simulink model "ART25_full_car_old"  (R2022a)
settings: Solver=ode1  StartTime=1  StopTime=10  FixedStep=0.0001  RelTol=1e-3
undefined symbols (not defined in the file or in its folder): canChannel, param, sim_TimeStep, vx0, yaw_rate0
libraries: canmsglib x5, slpidlib x4, canlib x2
settings Model: PacingRate=0.200000  Creator=jutri  LastModifiedBy=Usuario
settings SolverCC: PositivePriorityOrder=on
settings DataIOCC: SaveFormat=Array
settings OptimizationCC: BlockReduction=off  OptimizeBlockIOStorage=off
settings DebuggingCC: TasksWithSamePriorityMsg=none
settings HardwareCC: ProdBitPerLong=64  ProdHWDeviceType=Intel->x86-64 (Linux 64)
settings ModelReferenceCC: EnableRefExpFcnMdlSchedulingChecks=off  ModelReferenceNumInstancesAllowed=Single
settings RTWCC: Description=Simulink Desktop Real-Time  SystemTargetFile=sldrt.tlc  TemplateMakefile=sldrt.tmf  Toolchain=Simulink Real-Time Toolchain  BuildConfiguration=Faster Runs  TargetLang=C++  RTWCompilerOptimization=on
settings CodeAppCC: MaxIdLength=95
settings SimulinkDesktopRealTimeCC: TargetLibSuffix=_sldrt.a  TargetPreCompLibLocation=C:\Program Files\MATLAB\R2022a\toolbox\sldrt\lib\win64  TargetLangStandard=C++03 (ISO)

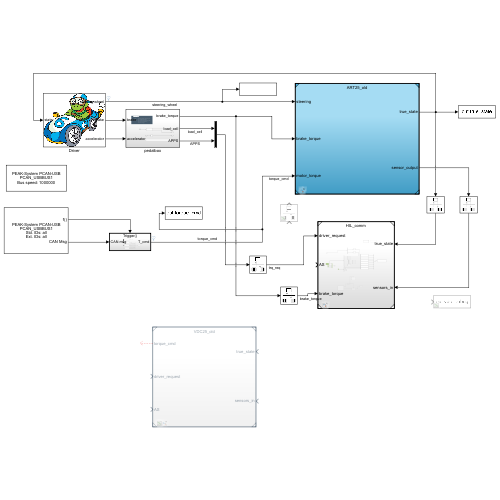
[thumbnail: Simulink's stored preview of the top-level diagram]
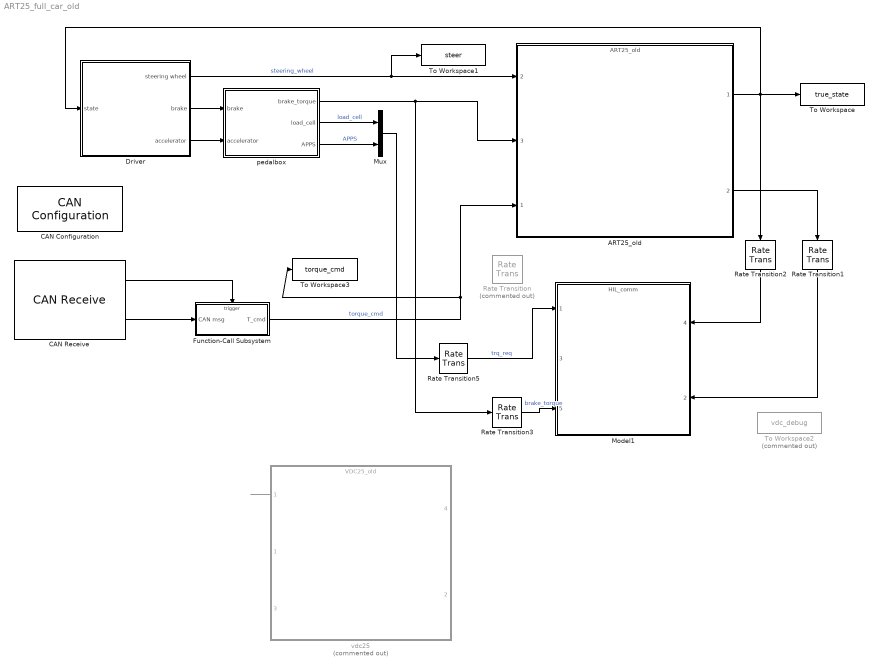
== system ART25_full_car_old ==
  ART25_old : ModelReference  ModelNameDialog=ART25_old.slx  SimulationMode=Normal  ModelReferenceVersion=1.103
      settings: PortSchema="{\"entries\":[{\"content\":{\"sides\":[{\"content\":{\"connectorIds\":[\"In2\",\"In3\",\"In1\"]},\"type\":\"ConnectorPlacement.EquallySpacedRectSide\",\"uuid\":\"34e73162-f48c-446a-824e-17dcc9cc6514\"},{\"content\":{\"connectorIds\":[\"Out1\",\"Out2\"],\"side\":\"RIGHT\"},\"type\":\"ConnectorPlacement.EquallySpacedRectSide\",\"uuid\":\"74737ed4-0958-463a-8e43-c11e4d3189aa\"},{\"content\":{\"side\":\"TOP\"},\"type\":\"ConnectorPlacement.EquallySpacedRectSide\",\"uuid\":\"42fc3775-e72e-4fbb-8cdc-9d9cf3c0f815\"}]},\"type\":\"ConnectorPlacement.EquallySpacedConnector\",\"uuid\":\"6e643428-a593-4a05-90a3-6bfae895b914\"}],\"packageUris\":[\"http://schema.mathworks.com/mf0/Connector/R2020b\"],\"version\":\"1.0\"}"
  CAN Configuration : canlib/CAN Configuration  BlockHandle=8.0004  Device=PEAK-System PCAN-USB (PCAN_USBBUS1)  DeviceMenu=PEAK-System PCAN-USB (PCAN_USBBUS1)  ObjConstructor=canChannel('PEAK-System', 'PCAN_USBBUS1')  BusSpeed=1000000  EnableBitParameters=off  AckMode=Normal
      settings: SourceProductBaseCode=VN
  CAN Receive : canlib/CAN Receive  BlockHandle=9.0004  Device=PEAK-System PCAN-USB (PCAN_USBBUS1)  DeviceMenu=PEAK-System PCAN-USB (PCAN_USBBUS1)  ObjConstructor=canChannel('PEAK-System', 'PCAN_USBBUS1')  EnableStandardIDsFilter=off  StdIDsCombo=Allow all  StandardIDs=0  EnableExtendedIDsFilter=off  ExtIDsCombo=Allow all  ExtendedIDs=0  SampleTime=sim_TimeStep  MsgsPerTimestep=all  InternalFilterUpdateStatus=on  BusOutput=off
      settings: SourceProductBaseCode=VN
  Driver : Subsystem
      mask Display: image('Driver_logo.jpeg');
  Function-Call Subsystem : Subsystem  TreatAsAtomicUnit=on
  Model1 : ModelReference  ModelNameDialog=HIL_comm.slx  SimulationMode=Normal  ModelReferenceVersion=1.270
      settings: PortSchema="{\"entries\":[{\"content\":{\"sides\":[{\"content\":{\"connectorIds\":[\"In1\",\"In3\",\"In5\"]},\"type\":\"ConnectorPlacement.EquallySpacedRectSide\",\"uuid\":\"04602d22-b9d7-40f7-b052-73f4143762fc\"},{\"content\":{\"connectorIds\":[\"In4\",\"In2\"],\"side\":\"RIGHT\"},\"type\":\"ConnectorPlacement.EquallySpacedRectSide\",\"uuid\":\"c5daacf6-0ad1-4531-a33a-b3ee5e66ed07\"},{\"content\":{\"connectorIds\":[],\"side\":\"TOP\"},\"type\":\"ConnectorPlacement.EquallySpacedRectSide\",\"uuid\":\"aa04230c-105f-45b7-b831-453931269445\"}]},\"type\":\"ConnectorPlacement.EquallySpacedConnector\",\"uuid\":\"55928aa8-a510-4f66-80b8-414931ecc3aa\"}],\"packageUris\":[\"http://schema.mathworks.com/mf0/Connector/R2020b\"],\"version\":\"1.0\"}"
  Mux : Mux  Inputs=2
  Rate Transition : RateTransition  Commented=on
  Rate Transition1 : RateTransition  Deterministic=off  OutPortSampleTime=vdc_TimeStep
  Rate Transition2 : RateTransition  OutPortSampleTime=vdc_TimeStep
  Rate Transition3 : RateTransition  OutPortSampleTime=vdc_TimeStep
  Rate Transition5 : RateTransition  OutPortSampleTime=vdc_TimeStep
  To Workspace : ToWorkspace  VariableName=true_state  SaveFormat=Structure With Time  SampleTime=-1
  To Workspace1 : ToWorkspace  VariableName=steer  SaveFormat=Structure  SampleTime=-1
  To Workspace2 : ToWorkspace  Commented=on  VariableName=vdc_debug  SaveFormat=Structure With Time  SampleTime=-1
  To Workspace3 : ToWorkspace  VariableName=torque_cmd  SaveFormat=Structure With Time  SampleTime=-1
  pedalbox : Subsystem
  vdc25 : ModelReference  Commented=on  ModelNameDialog=VDC25_old.slx  SimulationMode=Normal  ModelReferenceVersion=1.159
      settings: PortSchema="{\"entries\":[{\"content\":{\"sides\":[{\"content\":{\"connectorIds\":[\"Out1\",\"In1\",\"In3\"]},\"type\":\"ConnectorPlacement.EquallySpacedRectSide\",\"uuid\":\"da147370-b91a-4bb5-9c6b-40685e9dd617\"},{\"content\":{\"connectorIds\":[\"In4\",\"In2\"],\"side\":\"RIGHT\"},\"type\":\"ConnectorPlacement.EquallySpacedRectSide\",\"uuid\":\"d61eec38-a682-4bd1-95e6-e7fb713ea16a\"},{\"content\":{\"connectorIds\":[],\"side\":\"TOP\"},\"type\":\"ConnectorPlacement.EquallySpacedRectSide\",\"uuid\":\"c636197e-c055-4dae-9ca6-30a202bee6bf\"}]},\"type\":\"ConnectorPlacement.EquallySpacedConnector\",\"uuid\":\"636ba342-8237-45ef-8445-7b2704fdba3c\"}],\"packageUris\":[\"http://schema.mathworks.com/mf0/Connector/R2020b\"],\"version\":\"1.0\"}"
  wires:
  Driver/1(steering wheel) -> To Workspace1/1, ART25_old/2  "steering_wheel"
  ART25_old/2 -> Rate Transition1/1
  Driver/2(brake) -> pedalbox/1(brake)
  vdc25/1 -> ?
  ART25_old/1 -> Driver/1(state), Rate Transition2/1, To Workspace/1
  Driver/3(accelerator) -> pedalbox/2(accelerator)
  pedalbox/2(load_cell) -> Mux/1  "load_cell"
  pedalbox/3(APPS) -> Mux/2  "APPS"
  Rate Transition5/1 -> Model1/1  "trq_req"
  Rate Transition1/1 -> Model1/2
  Rate Transition2/1 -> Model1/4
  Mux/1 -> Rate Transition5/1
  CAN Receive/2 -> Function-Call Subsystem/1(CAN msg)
  CAN Receive/1 -> Function-Call Subsystem/Trigger
  Function-Call Subsystem/1(T_cmd) -> ART25_old/1, To Workspace3/1  "torque_cmd"
  Rate Transition3/1 -> Model1/5  "brake_torque"
  pedalbox/1(brake_torque) -> Rate Transition3/1, ART25_old/3

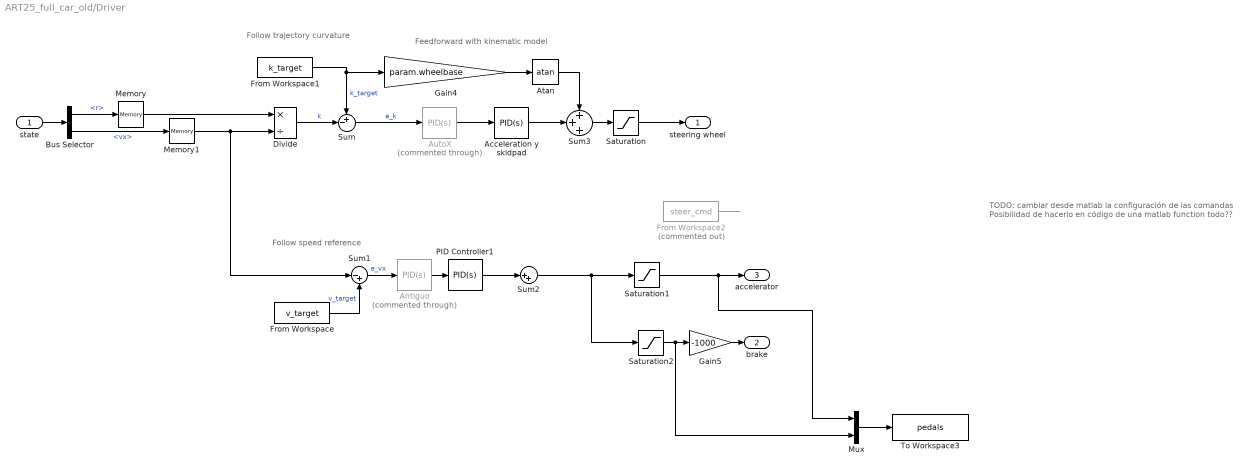
== system ART25_full_car_old/Driver ==
  note: TODO: cambiar desde matlab la configuración de las comandas
      | Posibilidad de hacerlo en código de una matlab function todo??
  note: Feedforward with kinematic model
  note: Follow trajectory curvature
  note: Follow speed reference
  state : Inport
  Acceleration y skidpad : slpidlib/PID Controller  Controller=PID  Form=Parallel  TimeDomain=Continuous-time  UseExternalTs=off  SampleTime=-1  IntegratorMethod=Forward Euler  FilterMethod=Forward Euler  ControllerParametersSource=internal  P=1  I=5  UseKiTs=off  D=0  N=1  UseFilter=on  TunerSelectOption=Transfer Function Based (PID Tuner App)  InitialConditionSource=internal  InitialConditionForIntegrator=0  InitialConditionForFilter=0  DifferentiatorICPrevScaledInput=0  ExternalReset=none  TrackingMode=off  Kt=1  LimitOutput=off  SatLimitsSource=internal  UpperSaturationLimit=inf  LowerSaturationLimit=-inf  LinearizeAsGain=on  AntiWindupMode=none  Kb=1  POutMin=[]  POutMax=[]  IOutMin=[]  IOutMax=[]  DOutMin=[]  DOutMax=[]  NOutMin=[]  NOutMax=[]  SumOutMin=[]  SumOutMax=[]  SaturationOutMin=[]  SaturationOutMax=[]  PParamMin=[]  PParamMax=[]  IParamMin=[]  IParamMax=[]  DParamMin=[]  DParamMax=[]  NParamMin=[]  NParamMax=[]  KbParamMin=[]  KbParamMax=[]  KtParamMin=[]  KtParamMax=[]  KbOutMin=[]  KbOutMax=[]  KtOutMin=[]  KtOutMax=[]  IntegratorOutMin=[]  IntegratorOutMax=[]  FilterOutMin=[]  FilterOutMax=[]  SumI1OutMin=[]  SumI1OutMax=[]  SumI2OutMin=[]  SumI2OutMax=[]  SumI3OutMin=[]  SumI3OutMax=[]  SumI4OutMin=[]  SumI4OutMax=[]  SumDOutMin=[]  SumDOutMax=[]  DifferentiatorOutMin=[]  DifferentiatorOutMax=[]  FilterDiffOutCoefMin=[]  FilterDiffOutCoefMax=[]  ReciprocalOutMin=[]  ReciprocalOutMax=[]  SumDenOutMin=[]  SumDenOutMax=[]  SumNumOutMin=[]  SumNumOutMax=[]  DivideOutMin=[]  DivideOutMax=[]  UdiffTsProdOutMin=[]  UdiffTsProdOutMax=[]  NTsProdOutMin=[]  NTsProdOutMax=[]  UintegralTsProdOutMin=[]  UintegralTsProdOutMax=[]  UngainTsProdOutMin=[]  UngainTsProdOutMax=[]  ClampingZeroOutDataTypeStr=Inherit: Inherit via back propagation  ClampingZeroOutMin=[]  ClampingZeroOutMax=[]  FilterDenConstantOutDataTypeStr=Inherit: Inherit via back propagation  FilterDenConstantOutMin=[]  FilterDenConstantOutMax=[]  PCopyOutDataTypeStr=Inherit: Inherit via back propagation  PCopyOutMin=[]  PCopyOutMax=[]  NCopyOutDataTypeStr=Inherit: Inherit via back propagation  NCopyOutMin=[]  NCopyOutMax=[]  IntegratorContinuousStateAttributes=''  IntegratorStateMustResolveToSignalObject=off  IntegratorRTWStateStorageClass=Auto  FilterContinuousStateAttributes=''  FilterStateMustResolveToSignalObject=off  FilterRTWStateStorageClass=Auto  ParallelPVariant=InternalParameters  IdealPVariant=Disabled  IVariant=InternalParameters  DVariant=InternalParameters  IntegratorVariant=Continuous  SatVariant=Disabled  AWVariant=Passthrough  PCopyVariant=Disabled  TRVariant=Disabled  FdbkBlocksVariant=Forward  IdealPFdbkVariant=Disabled  SatFdbkVariant=Disabled  DerivativeFilterVariant=ContFilter  NVariant=InternalParameters  NCopyVariant=Disabled  FilterICVariant=InternalICsFilter  IntegratorICVariant=InternalICs  ExternalResetVariant=Disabled  TRSumVariant=Passthrough  SumFdbkVariant=Disabled  SumVariant=Sum_PID  TsampFilterVariant=InternalTs  TsampNgainVariant=Passthrough  TsampIntegralVariant=Passthrough  ExternalSaturationOutDataTypeStr=Inherit: Same as second input  aMode=0
  Antiguo : slpidlib/PID Controller  Commented=through  Controller=PID  Form=Parallel  TimeDomain=Continuous-time  UseExternalTs=off  SampleTime=-1  IntegratorMethod=Forward Euler  FilterMethod=Forward Euler  ControllerParametersSource=internal  P=1  I=1  UseKiTs=off  D=0  N=10  UseFilter=on  TunerSelectOption=Transfer Function Based (PID Tuner App)  InitialConditionSource=internal  InitialConditionForIntegrator=0  InitialConditionForFilter=0  DifferentiatorICPrevScaledInput=0  ExternalReset=none  TrackingMode=off  Kt=1  LimitOutput=off  SatLimitsSource=internal  UpperSaturationLimit=inf  LowerSaturationLimit=-inf  LinearizeAsGain=on  AntiWindupMode=none  Kb=1  POutMin=[]  POutMax=[]  IOutMin=[]  IOutMax=[]  DOutMin=[]  DOutMax=[]  NOutMin=[]  NOutMax=[]  SumOutMin=[]  SumOutMax=[]  SaturationOutMin=[]  SaturationOutMax=[]  PParamMin=[]  PParamMax=[]  IParamMin=[]  IParamMax=[]  DParamMin=[]  DParamMax=[]  NParamMin=[]  NParamMax=[]  KbParamMin=[]  KbParamMax=[]  KtParamMin=[]  KtParamMax=[]  KbOutMin=[]  KbOutMax=[]  KtOutMin=[]  KtOutMax=[]  IntegratorOutMin=[]  IntegratorOutMax=[]  FilterOutMin=[]  FilterOutMax=[]  SumI1OutMin=[]  SumI1OutMax=[]  SumI2OutMin=[]  SumI2OutMax=[]  SumI3OutMin=[]  SumI3OutMax=[]  SumI4OutMin=[]  SumI4OutMax=[]  SumDOutMin=[]  SumDOutMax=[]  DifferentiatorOutMin=[]  DifferentiatorOutMax=[]  FilterDiffOutCoefMin=[]  FilterDiffOutCoefMax=[]  ReciprocalOutMin=[]  ReciprocalOutMax=[]  SumDenOutMin=[]  SumDenOutMax=[]  SumNumOutMin=[]  SumNumOutMax=[]  DivideOutMin=[]  DivideOutMax=[]  UdiffTsProdOutMin=[]  UdiffTsProdOutMax=[]  NTsProdOutMin=[]  NTsProdOutMax=[]  UintegralTsProdOutMin=[]  UintegralTsProdOutMax=[]  UngainTsProdOutMin=[]  UngainTsProdOutMax=[]  ClampingZeroOutDataTypeStr=Inherit: Inherit via back propagation  ClampingZeroOutMin=[]  ClampingZeroOutMax=[]  FilterDenConstantOutDataTypeStr=Inherit: Inherit via back propagation  FilterDenConstantOutMin=[]  FilterDenConstantOutMax=[]  PCopyOutDataTypeStr=Inherit: Inherit via back propagation  PCopyOutMin=[]  PCopyOutMax=[]  NCopyOutDataTypeStr=Inherit: Inherit via back propagation  NCopyOutMin=[]  NCopyOutMax=[]  IntegratorContinuousStateAttributes=''  IntegratorStateMustResolveToSignalObject=off  IntegratorRTWStateStorageClass=Auto  FilterContinuousStateAttributes=''  FilterStateMustResolveToSignalObject=off  FilterRTWStateStorageClass=Auto  ParallelPVariant=InternalParameters  IdealPVariant=Disabled  IVariant=InternalParameters  DVariant=InternalParameters  IntegratorVariant=Continuous  SatVariant=Disabled  AWVariant=Passthrough  PCopyVariant=Disabled  TRVariant=Disabled  FdbkBlocksVariant=Forward  IdealPFdbkVariant=Disabled  SatFdbkVariant=Disabled  DerivativeFilterVariant=ContFilter  NVariant=InternalParameters  NCopyVariant=Disabled  FilterICVariant=InternalICsFilter  IntegratorICVariant=InternalICs  ExternalResetVariant=Disabled  TRSumVariant=Passthrough  SumFdbkVariant=Disabled  SumVariant=Sum_PID  TsampFilterVariant=InternalTs  TsampNgainVariant=Passthrough  TsampIntegralVariant=Passthrough  ExternalSaturationOutDataTypeStr=Inherit: Same as second input  aMode=0
  Atan : Trigonometry  Operator=atan
  AutoX : slpidlib/PID Controller  Commented=through  Controller=PID  Form=Parallel  TimeDomain=Continuous-time  UseExternalTs=off  SampleTime=-1  IntegratorMethod=Forward Euler  FilterMethod=Forward Euler  ControllerParametersSource=internal  P=1  I=2  UseKiTs=off  D=0.4  N=500  UseFilter=on  TunerSelectOption=Transfer Function Based (PID Tuner App)  InitialConditionSource=internal  InitialConditionForIntegrator=0  InitialConditionForFilter=0  DifferentiatorICPrevScaledInput=0  ExternalReset=none  TrackingMode=off  Kt=1  LimitOutput=off  SatLimitsSource=internal  UpperSaturationLimit=inf  LowerSaturationLimit=-inf  LinearizeAsGain=on  AntiWindupMode=none  Kb=1  POutMin=[]  POutMax=[]  IOutMin=[]  IOutMax=[]  DOutMin=[]  DOutMax=[]  NOutMin=[]  NOutMax=[]  SumOutMin=[]  SumOutMax=[]  SaturationOutMin=[]  SaturationOutMax=[]  PParamMin=[]  PParamMax=[]  IParamMin=[]  IParamMax=[]  DParamMin=[]  DParamMax=[]  NParamMin=[]  NParamMax=[]  KbParamMin=[]  KbParamMax=[]  KtParamMin=[]  KtParamMax=[]  KbOutMin=[]  KbOutMax=[]  KtOutMin=[]  KtOutMax=[]  IntegratorOutMin=[]  IntegratorOutMax=[]  FilterOutMin=[]  FilterOutMax=[]  SumI1OutMin=[]  SumI1OutMax=[]  SumI2OutMin=[]  SumI2OutMax=[]  SumI3OutMin=[]  SumI3OutMax=[]  SumI4OutMin=[]  SumI4OutMax=[]  SumDOutMin=[]  SumDOutMax=[]  DifferentiatorOutMin=[]  DifferentiatorOutMax=[]  FilterDiffOutCoefMin=[]  FilterDiffOutCoefMax=[]  ReciprocalOutMin=[]  ReciprocalOutMax=[]  SumDenOutMin=[]  SumDenOutMax=[]  SumNumOutMin=[]  SumNumOutMax=[]  DivideOutMin=[]  DivideOutMax=[]  UdiffTsProdOutMin=[]  UdiffTsProdOutMax=[]  NTsProdOutMin=[]  NTsProdOutMax=[]  UintegralTsProdOutMin=[]  UintegralTsProdOutMax=[]  UngainTsProdOutMin=[]  UngainTsProdOutMax=[]  ClampingZeroOutDataTypeStr=Inherit: Inherit via back propagation  ClampingZeroOutMin=[]  ClampingZeroOutMax=[]  FilterDenConstantOutDataTypeStr=Inherit: Inherit via back propagation  FilterDenConstantOutMin=[]  FilterDenConstantOutMax=[]  PCopyOutDataTypeStr=Inherit: Inherit via back propagation  PCopyOutMin=[]  PCopyOutMax=[]  NCopyOutDataTypeStr=Inherit: Inherit via back propagation  NCopyOutMin=[]  NCopyOutMax=[]  IntegratorContinuousStateAttributes=''  IntegratorStateMustResolveToSignalObject=off  IntegratorRTWStateStorageClass=Auto  FilterContinuousStateAttributes=''  FilterStateMustResolveToSignalObject=off  FilterRTWStateStorageClass=Auto  ParallelPVariant=InternalParameters  IdealPVariant=Disabled  IVariant=InternalParameters  DVariant=InternalParameters  IntegratorVariant=Continuous  SatVariant=Disabled  AWVariant=Passthrough  PCopyVariant=Disabled  TRVariant=Disabled  FdbkBlocksVariant=Forward  IdealPFdbkVariant=Disabled  SatFdbkVariant=Disabled  DerivativeFilterVariant=ContFilter  NVariant=InternalParameters  NCopyVariant=Disabled  FilterICVariant=InternalICsFilter  IntegratorICVariant=InternalICs  ExternalResetVariant=Disabled  TRSumVariant=Passthrough  SumFdbkVariant=Disabled  SumVariant=Sum_PID  TsampFilterVariant=InternalTs  TsampNgainVariant=Passthrough  TsampIntegralVariant=Passthrough  ExternalSaturationOutDataTypeStr=Inherit: Same as second input  aMode=0
  Bus Selector : BusSelector  OutputSignals=r,vx
  Divide : Product  Inputs=*/
  From Workspace : FromWorkspace  VariableName=v_target
  From Workspace1 : FromWorkspace  VariableName=k_target
  From Workspace2 : FromWorkspace  Commented=on  VariableName=steer_cmd
  Gain4 : Gain  Gain=param.wheelbase
  Gain5 : Gain  Gain=-1000
  Memory : Memory  InitialCondition=yaw_rate0
  Memory1 : Memory  InitialCondition=vx0
  Mux : Mux  Inputs=2
  PID Controller1 : slpidlib/PID Controller  Controller=PID  Form=Parallel  TimeDomain=Continuous-time  UseExternalTs=off  SampleTime=-1  IntegratorMethod=Forward Euler  FilterMethod=Forward Euler  ControllerParametersSource=internal  P=1  I=1  UseKiTs=off  D=1.5  N=1  UseFilter=on  TunerSelectOption=Transfer Function Based (PID Tuner App)  InitialConditionSource=internal  InitialConditionForIntegrator=0  InitialConditionForFilter=0  DifferentiatorICPrevScaledInput=0  ExternalReset=none  TrackingMode=off  Kt=1  LimitOutput=on  SatLimitsSource=internal  UpperSaturationLimit=1  LowerSaturationLimit=-1  LinearizeAsGain=on  AntiWindupMode=clamping  Kb=1  POutMin=[]  POutMax=[]  IOutMin=[]  IOutMax=[]  DOutMin=[]  DOutMax=[]  NOutMin=[]  NOutMax=[]  SumOutMin=[]  SumOutMax=[]  SaturationOutMin=[]  SaturationOutMax=[]  PParamMin=[]  PParamMax=[]  IParamMin=[]  IParamMax=[]  DParamMin=[]  DParamMax=[]  NParamMin=[]  NParamMax=[]  KbParamMin=[]  KbParamMax=[]  KtParamMin=[]  KtParamMax=[]  KbOutMin=[]  KbOutMax=[]  KtOutMin=[]  KtOutMax=[]  IntegratorOutMin=[]  IntegratorOutMax=[]  FilterOutMin=[]  FilterOutMax=[]  SumI1OutMin=[]  SumI1OutMax=[]  SumI2OutMin=[]  SumI2OutMax=[]  SumI3OutMin=[]  SumI3OutMax=[]  SumI4OutMin=[]  SumI4OutMax=[]  SumDOutMin=[]  SumDOutMax=[]  DifferentiatorOutMin=[]  DifferentiatorOutMax=[]  FilterDiffOutCoefMin=[]  FilterDiffOutCoefMax=[]  ReciprocalOutMin=[]  ReciprocalOutMax=[]  SumDenOutMin=[]  SumDenOutMax=[]  SumNumOutMin=[]  SumNumOutMax=[]  DivideOutMin=[]  DivideOutMax=[]  UdiffTsProdOutMin=[]  UdiffTsProdOutMax=[]  NTsProdOutMin=[]  NTsProdOutMax=[]  UintegralTsProdOutMin=[]  UintegralTsProdOutMax=[]  UngainTsProdOutMin=[]  UngainTsProdOutMax=[]  ClampingZeroOutDataTypeStr=Inherit: Inherit via back propagation  ClampingZeroOutMin=[]  ClampingZeroOutMax=[]  FilterDenConstantOutDataTypeStr=Inherit: Inherit via back propagation  FilterDenConstantOutMin=[]  FilterDenConstantOutMax=[]  PCopyOutDataTypeStr=Inherit: Inherit via back propagation  PCopyOutMin=[]  PCopyOutMax=[]  NCopyOutDataTypeStr=Inherit: Inherit via back propagation  NCopyOutMin=[]  NCopyOutMax=[]  IntegratorContinuousStateAttributes=''  IntegratorStateMustResolveToSignalObject=off  IntegratorRTWStateStorageClass=Auto  FilterContinuousStateAttributes=''  FilterStateMustResolveToSignalObject=off  FilterRTWStateStorageClass=Auto  ParallelPVariant=InternalParameters  IdealPVariant=Disabled  IVariant=InternalParameters  DVariant=InternalParameters  IntegratorVariant=Continuous  SatVariant=Enabled  AWVariant=ContClampingParallel  PCopyVariant=Disabled  TRVariant=Disabled  FdbkBlocksVariant=Forward  IdealPFdbkVariant=Disabled  SatFdbkVariant=Disabled  DerivativeFilterVariant=ContFilter  NVariant=InternalParameters  NCopyVariant=Disabled  FilterICVariant=InternalICsFilter  IntegratorICVariant=InternalICs  ExternalResetVariant=Disabled  TRSumVariant=Passthrough  SumFdbkVariant=Disabled  SumVariant=Sum_PID  TsampFilterVariant=InternalTs  TsampNgainVariant=Passthrough  TsampIntegralVariant=Passthrough  ExternalSaturationOutDataTypeStr=Inherit: Same as second input  aMode=0
  Saturation : Saturate  UpperLimit=0.3  LowerLimit=-0.3
  Saturation1 : Saturate  UpperLimit=1  LowerLimit=0
  Saturation2 : Saturate  UpperLimit=0  LowerLimit=-1
  Sum : Sum  Inputs=+-|
  Sum1 : Sum  Inputs=|-+
  Sum2 : Sum  Inputs=|++
  Sum3 : Sum  Inputs=+++
  To Workspace3 : ToWorkspace  VariableName=pedals  SaveFormat=Structure With Time  SampleTime=-1
  steering wheel : Outport
  brake : Outport  Port=2
  accelerator : Outport  Port=3
  wires:
  PID Controller1/1 -> Sum2/1
  state/1 -> Bus Selector/1
  Bus Selector/1 -> Memory/1  "<r>"
  Bus Selector/2 -> Memory1/1  "<vx>"
  Divide/1 -> Sum/2  "k"
  Sum1/1 -> Antiguo/1  "e_vx"
  From Workspace1/1 -> Gain4/1, Sum/1  "k_target"
  Sum2/1 -> Saturation2/1, Saturation1/1
  Sum/1 -> AutoX/1  "e_k"
  Sum3/1 -> Saturation/1
  AutoX/1 -> Acceleration y skidpad/1
  Saturation/1 -> steering wheel/1
  From Workspace/1 -> Sum1/2  "v_target"
  Gain4/1 -> Atan/1
  Atan/1 -> Sum3/1
  Memory/1 -> Divide/1
  Memory1/1 -> Divide/2, Sum1/1
  From Workspace2/1 -> ?
  Saturation1/1 -> Mux/1, accelerator/1
  Saturation2/1 -> Mux/2, Gain5/1
  Gain5/1 -> brake/1
  Acceleration y skidpad/1 -> Sum3/2
  Antiguo/1 -> PID Controller1/1
  Mux/1 -> To Workspace3/1

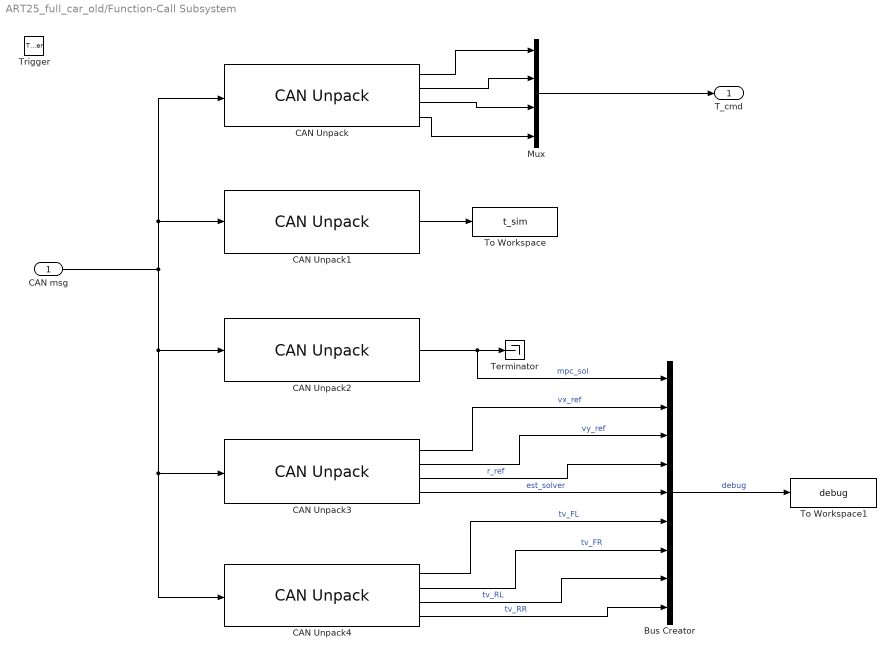
== system ART25_full_car_old/Function-Call Subsystem ==
  CAN msg : Inport
  Trigger : TriggerPort  TriggerType=function-call  VariantControl=(inherit)
  Bus Creator : BusCreator  Inputs=9
  CAN Unpack : canmsglib/CAN Unpack  MsgList=(none)  MsgName=Prueba  MsgIDType=Standard (11-bit identifier)  MsgIdentifier=0x100  MsgLength=8  SignalInfo={ 'Torque_FL', '0', '16', 'LE', 'signed', 'Standard', '0', '0.01', '0', '-Inf', 'Inf'; 'Torque_FR', '16', '16', 'LE', 'signed', 'Standard', '0', '0.01', '0', '-Inf', 'Inf'; 'Torque_RL', '32', '16', 'LE', 'signed', 'Standard', '0', '0.01', '0', '-Inf', 'Inf'; 'Torque_RR', '48', '16', 'LE', 'signed', 'Standard', '0', '0.01', '0', '-Inf', 'Inf' }  IDPort=off  TimestampPort=off  ErrorPort=off  RemotePort=off  LengthPort=off  StatusPort=off  ApplyMinMax=off
      settings: SourceProductBaseCode=XP,ME,VN
  CAN Unpack1 : canmsglib/CAN Unpack  MsgList=(none)  MsgName=Prueba  MsgIDType=Standard (11-bit identifier)  MsgIdentifier=0x101  MsgLength=2  SignalInfo={ 'T_sim', '0', '16', 'LE', 'unsigned', 'Standard', '0', '0.000001', '0', '-Inf', 'Inf' }  IDPort=off  TimestampPort=off  ErrorPort=off  RemotePort=off  LengthPort=off  StatusPort=off  ApplyMinMax=off
      settings: SourceProductBaseCode=XP,ME,VN
  CAN Unpack2 : canmsglib/CAN Unpack  MsgList=(none)  MsgName=Prueba  MsgIDType=Standard (11-bit identifier)  MsgIdentifier=0x102  MsgLength=2  SignalInfo={ 'mpc_sol', '0', '16', 'LE', 'signed', 'Standard', '0', '0.001', '0', '-Inf', 'Inf' }  IDPort=off  TimestampPort=off  ErrorPort=off  RemotePort=off  LengthPort=off  StatusPort=off  ApplyMinMax=off
      settings: SourceProductBaseCode=XP,ME,VN
  CAN Unpack3 : canmsglib/CAN Unpack  MsgList=(none)  MsgName=Prueba  MsgIDType=Standard (11-bit identifier)  MsgIdentifier=0x103  MsgLength=8  SignalInfo={ 'vx_ref', '0', '16', 'LE', 'signed', 'Standard', '0', '0.001', '0', '-Inf', 'Inf'; 'vy_ref', '16', '16', 'LE', 'signed', 'Standard', '0', '0.001', '0', '-Inf', 'Inf'; 'r_ref', '32', '16', 'LE', 'signed', 'Standard', '0', '0.0001', '0', '-Inf', 'Inf'; 'solver_est', '48', '16', 'LE', 'unsigned', 'Standard', '0', '1', '0', '-Inf', 'Inf' }  IDPort=off  TimestampPort=off  ErrorPort=off  RemotePort=off  LengthPort=off  StatusPort=off  ApplyMinMax=off
      settings: SourceProductBaseCode=XP,ME,VN
  CAN Unpack4 : canmsglib/CAN Unpack  MsgList=(none)  MsgName=Prueba  MsgIDType=Standard (11-bit identifier)  MsgIdentifier=0x104  MsgLength=8  SignalInfo={ 'Torque_FL', '0', '16', 'LE', 'signed', 'Standard', '0', '0.01', '0', '-Inf', 'Inf'; 'Torque_FR', '16', '16', 'LE', 'signed', 'Standard', '0', '0.01', '0', '-Inf', 'Inf'; 'Torque_RL', '32', '16', 'LE', 'signed', 'Standard', '0', '0.01', '0', '-Inf', 'Inf'; 'Torque_RR', '48', '16', 'LE', 'signed', 'Standard', '0', '0.01', '0', '-Inf', 'Inf' }  IDPort=off  TimestampPort=off  ErrorPort=off  RemotePort=off  LengthPort=off  StatusPort=off  ApplyMinMax=off
      settings: SourceProductBaseCode=XP,ME,VN
  Mux : Mux
  Terminator : Terminator
  To Workspace : ToWorkspace  VariableName=t_sim  SaveFormat=Structure With Time  SampleTime=-1
  To Workspace1 : ToWorkspace  VariableName=debug  SaveFormat=Structure With Time  SampleTime=-1
  T_cmd : Outport
  wires:
  CAN Unpack/1 -> Mux/1
  CAN Unpack/2 -> Mux/2
  Mux/1 -> T_cmd/1
  CAN Unpack/3 -> Mux/3
  CAN Unpack/4 -> Mux/4
  CAN Unpack1/1 -> To Workspace/1
  CAN Unpack2/1 -> Bus Creator/1, Terminator/1  "mpc_sol"
  CAN msg/1 -> CAN Unpack1/1, CAN Unpack/1, CAN Unpack4/1, CAN Unpack3/1, CAN Unpack2/1
  Bus Creator/1 -> To Workspace1/1  "debug"
  CAN Unpack3/1 -> Bus Creator/2  "vx_ref"
  CAN Unpack3/2 -> Bus Creator/3  "vy_ref"
  CAN Unpack3/3 -> Bus Creator/4  "r_ref"
  CAN Unpack3/4 -> Bus Creator/5  "est_solver"
  CAN Unpack4/1 -> Bus Creator/6  "tv_FL"
  CAN Unpack4/2 -> Bus Creator/7  "tv_FR"
  CAN Unpack4/3 -> Bus Creator/8  "tv_RL"
  CAN Unpack4/4 -> Bus Creator/9  "tv_RR"

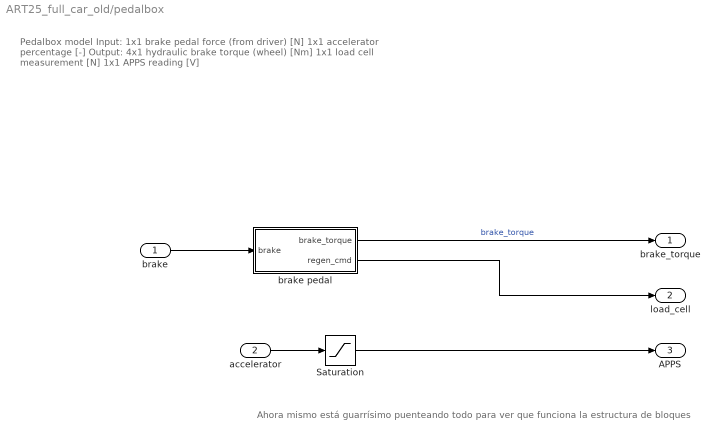
== system ART25_full_car_old/pedalbox ==
  note: Ahora mismo está guarrísimo puenteando todo para ver que funciona la estructura de bloques
  note: Pedalbox model
      |
      | Input: 1x1 brake pedal force (from driver) [N]
      | 1x1 accelerator percentage [-]
      |
      | Output: 4x1 hydraulic brake torque (wheel) [Nm]
      | 1x1 load cell measurement [N]
      | 1x1 APPS reading [V]
  brake : Inport
  accelerator : Inport  Port=2
  Saturation : Saturate  UpperLimit=1  LowerLimit=-1
  brake pedal : Subsystem
  brake_torque : Outport
  load_cell : Outport  Port=2
  APPS : Outport  Port=3
  wires:
  brake pedal/1(brake_torque) -> brake_torque/1  "brake_torque"
  brake/1 -> brake pedal/1(brake)
  accelerator/1 -> Saturation/1
  brake pedal/2(regen_cmd) -> load_cell/1
  Saturation/1 -> APPS/1

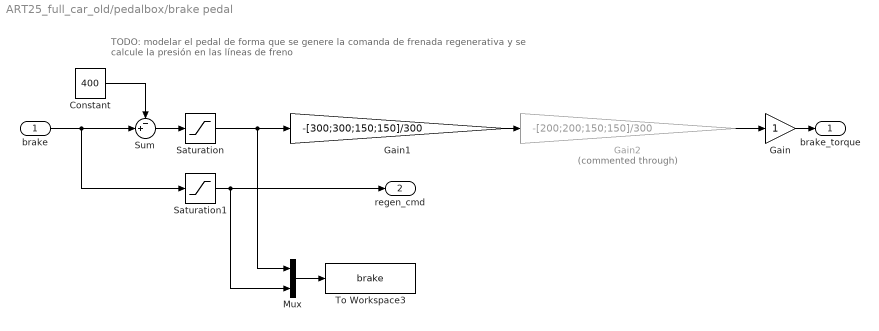
== system ART25_full_car_old/pedalbox/brake pedal ==
  note: TODO: modelar el pedal de forma que se genere la comanda de frenada regenerativa y se calcule la presión en las líneas de freno
  brake : Inport
  Constant : Constant  Value=400
  Gain : Gain
  Gain1 : Gain  Gain=-[300;300;150;150]/300
  Gain2 : Gain  Commented=through  Gain=-[200;200;150;150]/300
  Mux : Mux  Inputs=2
  Saturation : Saturate  UpperLimit=2000  LowerLimit=0
  Saturation1 : Saturate  UpperLimit=400  LowerLimit=0
  Sum : Sum  Inputs=-+|
  To Workspace3 : ToWorkspace  VariableName=brake  SaveFormat=Structure With Time  SampleTime=-1
  brake_torque : Outport
  regen_cmd : Outport  Port=2
  wires:
  Gain1/1 -> Gain2/1
  brake/1 -> Saturation1/1, Sum/2
  Sum/1 -> Saturation/1
  Constant/1 -> Sum/1
  Saturation1/1 -> Mux/2, regen_cmd/1
  Gain/1 -> brake_torque/1
  Gain2/1 -> Gain/1
  Mux/1 -> To Workspace3/1
  Saturation/1 -> Mux/1, Gain1/1
